simulink model "ccp_slave_demo"  (Simulink 7.3)
settings: Solver=ode3  SolverMode=SingleTasking  StartTime=0.0  StopTime=10.0  RelTol=1e-3
PreLoadFcn:
  | waijung.modelPreload; % Required for working with Waijung Blockset. Do not remove.
undefined symbols (not defined in the file): LQFP48, STM32F072CB
libraries: simulink x216, waijung_soft_i2c_lib x28, waijung_addon_module x12, stm32f0_flash_lib x10, stm32f0_can_lib x3, stm32f0_reset_lib x1, waijung_crc_lib x1, stm32f0_device_config_lib x1
(part 4 of 6)

== system ccp_slave_demo/CCP Handler/Command Processing/BUILD_CHKSUM/BUILD_CHKSUM Handler/Block Size ==
  In1 : Inport
  In2 : Inport  Port=2
  In3 : Inport  Port=3
  In4 : Inport  Port=4
  Bitwise Operator : simulink/Logic and Bit Operations/Bitwise Operator  logicop=OR  UseBitMask=off  NumInputPorts=4  BitMask=bin2dec('11011001')  BitMaskRealWorld=Stored Integer
  Data Type Conversion{1..4} (4 alike) : DataTypeConversion  OutDataTypeMode=uint32  OutDataType=fixdt(1, 16)  OutScaling=2^0  OutDataTypeStr=uint32
  Shift Arithmetic : simulink/Logic and Bit Operations/Shift Arithmetic  SystemSampleTime=-1  nBitShiftRight=-16  nBinPtShiftRight=0
  Shift Arithmetic1 : simulink/Logic and Bit Operations/Shift Arithmetic  SystemSampleTime=-1  nBitShiftRight=-8  nBinPtShiftRight=0
  Shift Arithmetic3 : simulink/Logic and Bit Operations/Shift Arithmetic  SystemSampleTime=-1  nBitShiftRight=-24  nBinPtShiftRight=0
  Size : Outport
  wires:
  In1/1 -> Data Type Conversion1/1
  In2/1 -> Data Type Conversion2/1
  In3/1 -> Data Type Conversion3/1
  In4/1 -> Data Type Conversion4/1
  Data Type Conversion2/1 -> Shift Arithmetic/1
  Data Type Conversion3/1 -> Shift Arithmetic1/1
  Data Type Conversion4/1 -> Bitwise Operator/4
  Data Type Conversion1/1 -> Shift Arithmetic3/1
  Shift Arithmetic/1 -> Bitwise Operator/2
  Shift Arithmetic1/1 -> Bitwise Operator/3
  Bitwise Operator/1 -> Size/1
  Shift Arithmetic3/1 -> Bitwise Operator/1

== system ccp_slave_demo/CCP Handler/Command Processing/BUILD_CHKSUM/BUILD_CHKSUM Handler/Subsystem ==
  In2 : Inport
  In3 : Inport  Port=2
  Enable : EnablePort
  While Iterator Subsystem : Subsystem  TreatAsAtomicUnit=on
  Out2 : Outport
  wires:
  In2/1 -> While Iterator Subsystem/1(Address)
  In3/1 -> While Iterator Subsystem/2(Size)
  While Iterator Subsystem/1(CRC) -> Out2/1

== system ccp_slave_demo/CCP Handler/Command Processing/BUILD_CHKSUM/BUILD_CHKSUM Handler/Subsystem1 ==
  In1 : Inport
  Bitwise Operator{1..4} (4 alike) : simulink/Logic and Bit Operations/Bitwise Operator  logicop=AND  UseBitMask=on  BitMask=255  BitMaskRealWorld=Stored Integer
  Data Type Conversion{,1..3} (4 alike) : DataTypeConversion  OutDataTypeMode=uint8  OutDataType=fixdt(1, 16)  OutScaling=2^0  OutDataTypeStr=uint8
  Shift Arithmetic : simulink/Logic and Bit Operations/Shift Arithmetic  SystemSampleTime=-1  nBitShiftRight=16  nBinPtShiftRight=0
  Shift Arithmetic1 : simulink/Logic and Bit Operations/Shift Arithmetic  SystemSampleTime=-1  nBitShiftRight=8  nBinPtShiftRight=0
  Shift Arithmetic4 : simulink/Logic and Bit Operations/Shift Arithmetic  SystemSampleTime=-1  nBitShiftRight=24  nBinPtShiftRight=0
  Out1 : Outport
  Out2 : Outport  Port=2
  Out3 : Outport  Port=3
  Out4 : Outport  Port=4
  wires:
  Shift Arithmetic/1 -> Bitwise Operator1/1
  Shift Arithmetic1/1 -> Bitwise Operator2/1
  Bitwise Operator4/1 -> Data Type Conversion/1
  Bitwise Operator1/1 -> Data Type Conversion1/1
  Bitwise Operator2/1 -> Data Type Conversion2/1
  Bitwise Operator3/1 -> Data Type Conversion3/1
  In1/1 -> Shift Arithmetic/1, Shift Arithmetic1/1, Bitwise Operator3/1, Shift Arithmetic4/1
  Data Type Conversion/1 -> Out1/1
  Data Type Conversion1/1 -> Out2/1
  Data Type Conversion2/1 -> Out3/1
  Data Type Conversion3/1 -> Out4/1
  Shift Arithmetic4/1 -> Bitwise Operator4/1

== system ccp_slave_demo/CCP Handler/Command Processing/CLEAR_MEMORY/CLEAR_MEMORY Handler/Block Size ==
  In1 : Inport
  In2 : Inport  Port=2
  In3 : Inport  Port=3
  In4 : Inport  Port=4
  Bitwise Operator : simulink/Logic and Bit Operations/Bitwise Operator  logicop=OR  UseBitMask=off  NumInputPorts=4  BitMask=bin2dec('11011001')  BitMaskRealWorld=Stored Integer
  Data Type Conversion{1..4} (4 alike) : DataTypeConversion  OutDataTypeMode=uint32  OutDataType=fixdt(1, 16)  OutScaling=2^0  OutDataTypeStr=uint32
  Shift Arithmetic : simulink/Logic and Bit Operations/Shift Arithmetic  SystemSampleTime=-1  nBitShiftRight=-16  nBinPtShiftRight=0
  Shift Arithmetic1 : simulink/Logic and Bit Operations/Shift Arithmetic  SystemSampleTime=-1  nBitShiftRight=-8  nBinPtShiftRight=0
  Shift Arithmetic3 : simulink/Logic and Bit Operations/Shift Arithmetic  SystemSampleTime=-1  nBitShiftRight=-24  nBinPtShiftRight=0
  Size : Outport
  wires:
  In1/1 -> Data Type Conversion1/1
  In2/1 -> Data Type Conversion2/1
  In3/1 -> Data Type Conversion3/1
  In4/1 -> Data Type Conversion4/1
  Data Type Conversion2/1 -> Shift Arithmetic/1
  Data Type Conversion3/1 -> Shift Arithmetic1/1
  Data Type Conversion4/1 -> Bitwise Operator/4
  Data Type Conversion1/1 -> Shift Arithmetic3/1
  Shift Arithmetic/1 -> Bitwise Operator/2
  Shift Arithmetic1/1 -> Bitwise Operator/3
  Bitwise Operator/1 -> Size/1
  Shift Arithmetic3/1 -> Bitwise Operator/1

== system ccp_slave_demo/CCP Handler/Command Processing/CLEAR_MEMORY/CLEAR_MEMORY Handler/Flash Erase ==
  Address : Inport
  Size : Inport  Port=2
  Enable : EnablePort
  Terminator4 : Terminator
  While Iterator Subsystem : Subsystem  TreatAsAtomicUnit=on
  wires:
  While Iterator Subsystem/1(Sta) -> Terminator4/1
  Address/1 -> While Iterator Subsystem/1(Address)
  Size/1 -> While Iterator Subsystem/2(Size)

== system ccp_slave_demo/CCP Handler/Command Processing/DNLOAD/DNLOAD_6/DOWNLOAD/DOWNLOAD_6 Handler/Subsystem1 ==
  In1 : Inport
  Bitwise Operator{1..4} (4 alike) : simulink/Logic and Bit Operations/Bitwise Operator  logicop=AND  UseBitMask=on  BitMask=255  BitMaskRealWorld=Stored Integer
  Data Type Conversion{,1..3} (4 alike) : DataTypeConversion  OutDataTypeMode=uint8  OutDataType=fixdt(1, 16)  OutScaling=2^0  OutDataTypeStr=uint8
  Shift Arithmetic : simulink/Logic and Bit Operations/Shift Arithmetic  SystemSampleTime=-1  nBitShiftRight=16  nBinPtShiftRight=0
  Shift Arithmetic1 : simulink/Logic and Bit Operations/Shift Arithmetic  SystemSampleTime=-1  nBitShiftRight=8  nBinPtShiftRight=0
  Shift Arithmetic3 : simulink/Logic and Bit Operations/Shift Arithmetic  SystemSampleTime=-1  nBitShiftRight=24  nBinPtShiftRight=0
  Out1 : Outport
  Out2 : Outport  Port=2
  Out3 : Outport  Port=3
  Out4 : Outport  Port=4
  wires:
  Shift Arithmetic/1 -> Bitwise Operator1/1
  Shift Arithmetic1/1 -> Bitwise Operator2/1
  Bitwise Operator4/1 -> Data Type Conversion/1
  Bitwise Operator1/1 -> Data Type Conversion1/1
  Bitwise Operator2/1 -> Data Type Conversion2/1
  Bitwise Operator3/1 -> Data Type Conversion3/1
  In1/1 -> Shift Arithmetic/1, Shift Arithmetic1/1, Bitwise Operator3/1, Shift Arithmetic3/1
  Data Type Conversion/1 -> Out1/1
  Data Type Conversion1/1 -> Out2/1
  Data Type Conversion2/1 -> Out3/1
  Data Type Conversion3/1 -> Out4/1
  Shift Arithmetic3/1 -> Bitwise Operator4/1

== system ccp_slave_demo/CCP Handler/Command Processing/DNLOAD/DNLOAD_6/DOWNLOAD/DOWNLOAD_6 Handler/Write DOWNLOAD ==
  Offset : Inport
  Data : Inport  Port=2
  Size : Inport  Port=3
  Enable : EnablePort
  Volatile Data Array Write : waijung_addon_module/Data Storage/Volatile Data Array Write  conf=Write  specificaddress=off  storagename=CONTROL  memoryaddress=hex2dec('64000000')  storagetype=uint8  datasize=120*160*3  varname=VolatileDataArray_CONTROL  datatype=uint8  datacount=5  variablesize=on  portpinstr=0  sampletime=inf  blockid=CCPHandlerCommandProcessingDNLOADDNLOAD_6DOWNLOADDOWNLOAD_6HandlerWriteDOWNLOADVolatileDataArrayWrite  inputporttype=[7 3 7]  inputportwidth=[1 5 1 ]  inputportlabel={'Offset', 'Data','Size'}  outputporttype=[]  outputportwidth=[]  outputportlabel={}  compat=0  optionstring="[\"CONTROL\",\"uint8\",\"256\",\"VolatileDataArray_CONTROL\",\"uint8_t\",\"uint8\",\"uint8_t\",\"5\",\"Param1\"]"
  wires:
  Size/1 -> Volatile Data Array Write/3
  Offset/1 -> Volatile Data Array Write/1
  Data/1 -> Volatile Data Array Write/2

== system ccp_slave_demo/CCP Handler/Command Processing/DNLOAD/DNLOAD_6/DOWNLOAD/DOWNLOAD_6 Handler/Write DOWNLOAD_6 ==
  Offset : Inport
  Data : Inport  Port=2
  Enable : EnablePort
  Volatile Data Array Write : waijung_addon_module/Data Storage/Volatile Data Array Write  conf=Write  specificaddress=off  storagename=CONTROL  memoryaddress=hex2dec('64000000')  storagetype=uint8  datasize=120*160*3  varname=VolatileDataArray_CONTROL  datatype=uint8  datacount=6  variablesize=off  portpinstr=0  sampletime=inf  blockid=CCPHandlerCommandProcessingDNLOADDNLOAD_6DOWNLOADDOWNLOAD_6HandlerWriteDOWNLOAD_6VolatileDataArrayWrite  inputporttype=[7 3]  inputportwidth=[1 6]  inputportlabel={'Offset', 'Data'}  outputporttype=[]  outputportwidth=[]  outputportlabel={}  compat=0  optionstring="[\"CONTROL\",\"uint8\",\"256\",\"VolatileDataArray_CONTROL\",\"uint8_t\",\"uint8\",\"uint8_t\",\"6\",\"Param1\"]"
  wires:
  Data/1 -> Volatile Data Array Write/2
  Offset/1 -> Volatile Data Array Write/1

== system ccp_slave_demo/CCP Handler/Command Processing/PROGRAM/ PROGRAM_6/PROGRAM/PROGRAM_6 Handler/EEPROM Program ==
  Offset : Inport
  Data(6) : Inport  Port=2
  Enable : EnablePort
  Compare To Constant : simulink/Logic and Bit Operations/Compare To Constant  SystemSampleTime=-1  relop===  const=1  LogicOutDataTypeMode=uint8  ZeroCross=off
  Compare To Constant1 : simulink/Logic and Bit Operations/Compare To Constant  SystemSampleTime=-1  relop===  const=2  LogicOutDataTypeMode=uint8  ZeroCross=off
  Compare To Constant2 : simulink/Logic and Bit Operations/Compare To Constant  SystemSampleTime=-1  relop===  const=3  LogicOutDataTypeMode=uint8  ZeroCross=off
  Compare To Constant3 : simulink/Logic and Bit Operations/Compare To Constant  SystemSampleTime=-1  relop===  const=4  LogicOutDataTypeMode=uint8  ZeroCross=off
  Compare To Constant4 : simulink/Logic and Bit Operations/Compare To Constant  SystemSampleTime=-1  relop===  const=5  LogicOutDataTypeMode=uint8  ZeroCross=off
  Constant2 : Constant  Value=hex2dec('A0')  OutDataTypeMode=uint8  OutDataType=fixdt(1, 16)  OutScaling=2^0  OutDataTypeStr=uint8
  Data Type Conversion : DataTypeConversion  OutDataType=fixdt(1, 16)  OutScaling=2^0
  Demux : Demux  Outputs=6
  Logical Operator{,1..4} (5 alike) : Logic  AllPortsSameDT=off  OutDataTypeMode=boolean  LogicDataType=fixdt(0, 8)  OutDataTypeStr=boolean
  Logical Operator5 : Logic  Operator=OR  Inputs=5  AllPortsSameDT=off  OutDataTypeMode=boolean  LogicDataType=fixdt(0, 8)  OutDataTypeStr=boolean
  Subsystem : Subsystem
  Subsystem1 : Subsystem
  Subsystem2 : Subsystem
  Subsystem3 : Subsystem
  Subsystem4 : Subsystem
  Success : Outport  OutDataType=fixdt(1, 16)  OutScaling=2^0
  wires:
  Data(6)/1 -> Demux/1
  Offset/1 -> Data Type Conversion/1
  Constant2/1 -> Subsystem/1(SlaveAddr), Subsystem1/1(SlaveAddr), Subsystem2/1(SlaveAddr), Subsystem3/1(SlaveAddr), Subsystem4/1(SlaveAddr)
  Data Type Conversion/1 -> Subsystem/2(Offset), Subsystem1/2(Offset), Subsystem2/2(Offset), Subsystem3/2(Offset), Subsystem4/2(Offset)
  Demux/2 -> Subsystem/3(D0), Subsystem1/3(D0), Subsystem2/3(D0), Subsystem3/3(D0), Subsystem4/3(D0)
  Demux/1 -> Compare To Constant/1, Compare To Constant1/1, Compare To Constant2/1, Compare To Constant3/1, Compare To Constant4/1
  Compare To Constant/1 -> Subsystem/Enable, Logical Operator/1
  Compare To Constant1/1 -> Subsystem1/Enable, Logical Operator1/1
  Demux/3 -> Subsystem1/4(D1), Subsystem2/4(D1), Subsystem3/4(D1), Subsystem4/4(D1)
  Compare To Constant2/1 -> Subsystem2/Enable, Logical Operator2/1
  Demux/4 -> Subsystem2/5(D2), Subsystem3/5(D2), Subsystem4/5(D2)
  Compare To Constant3/1 -> Subsystem3/Enable, Logical Operator3/1
  Demux/5 -> Subsystem3/6(D3), Subsystem4/6(D3)
  Demux/6 -> Subsystem4/7(D4)
  Compare To Constant4/1 -> Subsystem4/Enable, Logical Operator4/1
  Subsystem/1(Success) -> Logical Operator/2
  Subsystem1/1(Success) -> Logical Operator1/2
  Subsystem2/1(Success) -> Logical Operator2/2
  Subsystem3/1(Success) -> Logical Operator3/2
  Subsystem4/1(Success) -> Logical Operator4/2
  Logical Operator/1 -> Logical Operator5/1
  Logical Operator4/1 -> Logical Operator5/5
  Logical Operator3/1 -> Logical Operator5/4
  Logical Operator2/1 -> Logical Operator5/3
  Logical Operator1/1 -> Logical Operator5/2
  Logical Operator5/1 -> Success/1

== system ccp_slave_demo/CCP Handler/Command Processing/PROGRAM/ PROGRAM_6/PROGRAM/PROGRAM_6 Handler/EEPROM Program 6 ==
  Offset : Inport
  Data(6) : Inport  Port=2
  Enable : EnablePort
  Constant2 : Constant  Value=hex2dec('A0')  OutDataTypeMode=uint8  OutDataType=fixdt(1, 16)  OutScaling=2^0  OutDataTypeStr=uint8
  Data Type Conversion : DataTypeConversion  OutDataType=fixdt(1, 16)  OutScaling=2^0
  Demux : Demux  Outputs=6
  MEM_FLASH : simulink/Logic and Bit Operations/Compare To Constant  SystemSampleTime=-1  relop===  const=0  LogicOutDataTypeMode=uint8  ZeroCross=off
  Soft I2C Master Read/Write : waijung_soft_i2c_lib/Soft I2C Master Read//Write  conf=ReadWrite  targetname=stm32f0  module=1  transfer=Blocking  clk=100  timeout=25  sdapins={'A4','A6'}  sclpins='A5'  writecount=7  readcount=0  waittime=5  forcestop=off  portpinstr=0  sampletime=inf  blockid=CCPHandlerCommandProcessingPROGRAMPROGRAM_6PROGRAMPROGRAM_6HandlerEEPROMProgram6SoftI2CMasterReadWrite  inputporttype=[3 3 3 3 3 3 3 3]  inputportwidth=[]  inputportlabel={'SlvAddr' 'Wr0 (uint8)' 'Wr1 (uint8)' 'Wr2 (uint8)' 'Wr3 (uint8)' 'Wr4 (uint8)' 'Wr5 (uint8)' 'Wr6 (uint8)'}  outputporttype=[3]  outputportwidth=[1]  outputportlabel={'Status'}  compat=0  optionstring="[\"1\",\"7\",\"0\",\"5\",\"off\",\"1\"]"
  Success : Outport  OutDataType=fixdt(1, 16)  OutScaling=2^0
  wires:
  Data(6)/1 -> Demux/1
  Constant2/1 -> Soft I2C Master Read/Write/1
  Offset/1 -> Data Type Conversion/1
  Data Type Conversion/1 -> Soft I2C Master Read/Write/2
  Demux/1 -> Soft I2C Master Read/Write/3
  Demux/2 -> Soft I2C Master Read/Write/4
  Demux/3 -> Soft I2C Master Read/Write/5
  Demux/4 -> Soft I2C Master Read/Write/6
  Demux/5 -> Soft I2C Master Read/Write/7
  Demux/6 -> Soft I2C Master Read/Write/8
  Soft I2C Master Read/Write/1 -> MEM_FLASH/1
  MEM_FLASH/1 -> Success/1

== system ccp_slave_demo/CCP Handler/Command Processing/PROGRAM/ PROGRAM_6/PROGRAM/PROGRAM_6 Handler/Flash Program ==
  Offset : Inport
  Data(6) : Inport  Port=2
  Enable : EnablePort
  Compare To Constant : simulink/Logic and Bit Operations/Compare To Constant  SystemSampleTime=-1  relop===  const=2  LogicOutDataTypeMode=uint8  ZeroCross=off
  Compare To Constant1 : simulink/Logic and Bit Operations/Compare To Constant  SystemSampleTime=-1  relop===  const=4  LogicOutDataTypeMode=uint8  ZeroCross=off
  Demux : Demux  Outputs=6
  Logical Operator1 : Logic  AllPortsSameDT=off  OutDataTypeMode=boolean  LogicDataType=fixdt(0, 8)  OutDataTypeStr=boolean
  Logical Operator2 : Logic  Operator=OR  AllPortsSameDT=off  OutDataTypeMode=boolean  LogicDataType=fixdt(0, 8)  OutDataTypeStr=boolean
  Logical Operator4 : Logic  AllPortsSameDT=off  OutDataTypeMode=boolean  LogicDataType=fixdt(0, 8)  OutDataTypeStr=boolean
  Subsystem : Subsystem
  Subsystem1 : Subsystem
  Terminator1 : Terminator
  UART Tx : S-Function  FunctionName=stm32f0_uart  Parameters=conf,inputporttype,inputportwidth,outputporttype,outputportwidth,asciiheader,optionstring,headerstring,terminatorstring,asciidatatypestring,sampletime,blockid  EnableBusSupport=off  mask(stm32f0_uart){conf=Tx, uartmodule=1, baudrate=115200, databits=8, parity=No, stopbit=1, remaptxpin=A9, remaprxpin=A10, flowcontrol=None, remapctspin=Not used, remaprtspin=Not used, advanceoptions=off, rxbuffersize=64, txbuffersize=64, transfer=Non-Blocking, packetmode=Ascii, binheader='7E 7E', binterminator='03 03', porttype_double=0, porttype_single=0, porttype_int8=0, porttype_uint8=0, porttype_int16=0, porttype_uint16=0, porttype_int32=0, porttype_uint32=2, asciiformat='Program6: 0x%X, sta=%u,%u', rx_asciiterminator=CR (0x0D - "\r"), tx_asciiterminator=CRLF (0x0D 0x0A - "\r\n"), storagename=<empty>, varname=, asciiheader=Program6: 0x%X, sta=%u,%u\r\n, sampletime=inf, enablecustomportlabel=off, cinputportlabel=de, coutputportlabel=fff,ff,sdfsd, portpinstr=0, blockid=CCPHandlerCommandProcessingPROGRAMPROGRAM_6PROGRAMPROGRAM_6HandlerFlashProgramUARTTx, inputporttype=[ -1 -1 -1], inputportwidth=[], inputportlabel={ '%X' '%u' '%u'}, outputporttype=[], outputportwidth=[], outputportlabel={}, compat=0, optionstring=["1", "1", "A", "9", "1", "A", "10", "0", "*", "*", "0", "*", "*", "1", "1", "", "", "115200", "8", "No", "1", "None", "3", "2", "64", "64", "Ascii", "Non-Blocking", ""], headerstring=[], terminatorstring=["13","10"], asciidatatypestring=["uint32_t","uint32_t","uint32_t"], lastmodule=1}
      mask prompts: conf "Configuration"; uartmodule "UART Module"; baudrate "Baud rate (bps)"; databits "Data bits"; stopbit "Stop bit"; remaptxpin "Tx pin"; remaprxpin "Rx pin"; flowcontrol "Hardware flow control"; remapctspin "HW Flow control, CTS Pin"; remaprtspin "HW Flow control, RTS Pin"; advanceoptions "Advance options"; rxbuffersize "Rx buffer size (bytes)"; txbuffersize "Tx buffer size (bytes)"; packetmode "Packet mode"; binheader "Binary header (example: '7E 7E')"; binterminator "Binary terminator (example: '03 03')"; porttype_double "Number of data port, type DOUBLE"; porttype_single "Number of data port, type SINGLE"; porttype_int8 "Number of data port, type INT8"; porttype_uint8 "Number of data port, type UINT8"; porttype_int16 "Number of data port, type INT16"; porttype_uint16 "Number of data port, type UINT16"; porttype_int32 "Number of data port, type INT32"; porttype_uint32 "Number of data port, type UINT32"; asciiformat "Ascii format"; rx_asciiterminator "End of packet"; tx_asciiterminator "End of packet"; storagename "Buffer"; varname "Var name"; asciiheader "Ascii header (printf format)"; sampletime "Sample time (sec)"; enablecustomportlabel "Enable custom port labels (Ex. In1, In2, In3)"; cinputportlabel "Custom input port labels (Ex. In1, In2, In3)"; coutputportlabel "Custom output port labels (Ex. Out1, Out2, Out3)"; portpinstr "Port Pin String"; blockid "Block ID"; inputporttype "Input Port Type"; inputportwidth "Input Port Width"; inputportlabel "Input Port Label"; outputporttype "Output Port Type"; outputportwidth "Output Port Width"; outputportlabel "Output port label"; compat "Compatibility (Reserved for future use)"; optionstring "String(s) to be passed to TLC"; lastmodule "Last module selected"
      mask help:
      | UART Module
      |  - Select module corresponding to "UART Setup" block.
      | Transfer
      |  - Blocking: after write DMA buffer, the block wait until buffer empty.
      |  - Non-Blocking: the block will not wait for buffer empty.
      | Packet mode:
      |  - Ascii: sending data is ascii, Ascii format + End of packet.
      |  - Binary: sending data is binary format, Header + Data + Terminator
      |  - String Buffer: Volatile Data Storage variable name as sending data.
      | Ascii format:
      |  - %U, %I, %D, %O, %X, %u, %i, %d, %o, %x: Uint32
      |  - %E, %G, %F, %e, %g, %f: Single
      |  - %C, %c: Int8
      |  - %S, %s: (char *), this port is output of Volatile Data Storage Read block, which data type is string.
      mask init:
      | stm32f0_uart_callback('init');
      mask Help: web(fullfile(waijungdocroot,'stm32f0_uart_tx.htm'), '-browser')
      mask StyleString: popup(Setup|Tx|Rx),popup(1|2|3|4),edit,popup(8),popup(No|Odd|Even),popup(0.5|1|1.5|2),popup(Not used|A9|B6),popup(Not used|A10|B7),popup(None|RTS|CTS|RTS/CTS),popup(Not used|A11),popup(Not used|A12),checkbox,popup(16|32|64|128|256|512),popup(16|32|64|128|256|512),popup(Blocking|Non-Blocking),popup(Ascii|Binary|String Buffer),edit,edit,edit,edit,edit,edit,edit,edit,edit,edit,edit,popup(CR (0x0D - "\r")|LF (0x0A - "\n")|CRLF (0x0D 0x0A - "\r\n")),popup(CR (0x0D - "\r")|LF (0x0A - "\n")|CRLF (0x0D 0x0A - "\r\n")|None),popup(<empty>),edit,edit,edit,checkbox,edit,edit,edit,edit,edit,edit,edit,edit,edit,edit,edit,edit,edit,edit,edit,edit
      mask CallbackString: stm32f0_uart_callback('conf');|stm32f0_uart_callback('uartmodule');|||||||stm32f0_uart_callback('flowcontrol');|||stm32f0_uart_callback('advanceoptions');|||stm32f0_uart_callback('conf');|stm32f0_uart_callback('conf');|stm32f0_uart_callback('binheader');|stm32f0_uart_callback('binterminator');|||||||||stm32f0_uart_callback('asciiformat');|||stm32f0_uart_callback('storagename');|||stm32f0_uart_callback('sampletime');|stm32f0_uart_callback('enablecustomportlabel');|stm32f0_uart_callback('conf');|stm32f0_uart_callback('conf');||stm32f0_uart_callback('blockid');||||||||||||
      mask Display: text(0.95, 0.5, 'Module: USART1_Tx\nPacket: Ascii\nTransfer: Non-Blocking\nTs (sec): 0.01','ver','middle','hor','right'); port_label('input', 1,'%X'); port_label('input', 2,'%u'); port_label('input', 3,'%u');
  Success : Outport  OutDataType=fixdt(1, 16)  OutScaling=2^0
  wires:
  Data(6)/1 -> Demux/1
  Offset/1 -> Subsystem/1(Addr), Subsystem1/1(Addr), UART Tx/1
  Demux/2 -> Subsystem/2(In3), Subsystem1/2(In3)
  Demux/3 -> Subsystem/3(In4), Subsystem1/3(In4)
  Demux/1 -> Compare To Constant/1, Compare To Constant1/1
  Compare To Constant/1 -> Subsystem/Enable, Logical Operator4/1
  Compare To Constant1/1 -> Subsystem1/Enable, Logical Operator1/1
  Demux/4 -> Subsystem1/4(In1)
  Demux/5 -> Subsystem1/5(In2)
  Demux/6 -> Terminator1/1
  Subsystem/1(Success) -> Logical Operator4/2
  Subsystem1/1(Success) -> Logical Operator1/2
  Logical Operator4/1 -> Logical Operator2/1, UART Tx/2
  Logical Operator1/1 -> Logical Operator2/2, UART Tx/3
  Logical Operator2/1 -> Success/1

== system ccp_slave_demo/CCP Handler/Command Processing/PROGRAM/ PROGRAM_6/PROGRAM/PROGRAM_6 Handler/Flash Program 6 ==
  Offset : Inport
  Data(6) : Inport  Port=2
  Enable : EnablePort
  Add : Sum  OutDataType=fixdt(1, 16)  OutScaling=2^-10
  Constant : Constant  Value=2  OutDataTypeMode=uint32  OutDataType=fixdt(1, 16)  OutScaling=2^0  OutDataTypeStr=uint32
  Demux2 : Demux  Outputs=6
  FLASH Write : stm32f0_flash_lib/FLASH Write  conf=Write  startaddress=0x8011000  pagesize=2k  datatype=uint16  enablestatus=on  sampletime=inf  filename='ccp_slave_demo.flash'  enablecustomportlabel=off  cinputportlabel=0  portpinstr=0  blockid=CCPHandlerCommandProcessingPROGRAMPROGRAM_6PROGRAMPROGRAM_6HandlerFlashProgram6FLASHWrite  inputporttype=[7 5]  inputportwidth=[]  inputportlabel={'Offset','Data (uint16)'}  outputporttype=[3]  outputportwidth=[]  outputportlabel={'Status'}  compat=0  optionstring="[\"8011000\",\"0\"]"
  FLASH Write1 : stm32f0_flash_lib/FLASH Write  conf=Write  startaddress=0x8011000  pagesize=2k  datatype=uint32  enablestatus=on  sampletime=inf  filename='ccp_slave_demo.flash'  enablecustomportlabel=off  cinputportlabel=0  portpinstr=0  blockid=CCPHandlerCommandProcessingPROGRAMPROGRAM_6PROGRAMPROGRAM_6HandlerFlashProgram6FLASHWrite1  inputporttype=[7 7]  inputportwidth=[]  inputportlabel={'Offset','Data (uint32)'}  outputporttype=[3]  outputportwidth=[]  outputportlabel={'Status'}  compat=0  optionstring="[\"8011000\",\"0\"]"
  FLASH_COMPLETE : simulink/Logic and Bit Operations/Compare To Constant  SystemSampleTime=-1  relop===  const=4  LogicOutDataTypeMode=uint8  ZeroCross=off
  FLASH_COMPLETE1 : simulink/Logic and Bit Operations/Compare To Constant  SystemSampleTime=-1  relop===  const=4  LogicOutDataTypeMode=uint8  ZeroCross=off
  Logical Operator : Logic  AllPortsSameDT=off  OutDataTypeMode=boolean  LogicDataType=fixdt(0, 8)  OutDataTypeStr=boolean
  Subsystem : Subsystem
  Subsystem1 : Subsystem
  UART Tx : S-Function  FunctionName=stm32f0_uart  Parameters=conf,inputporttype,inputportwidth,outputporttype,outputportwidth,asciiheader,optionstring,headerstring,terminatorstring,asciidatatypestring,sampletime,blockid  EnableBusSupport=off  mask(stm32f0_uart){conf=Tx, uartmodule=1, baudrate=115200, databits=8, parity=No, stopbit=1, remaptxpin=A9, remaprxpin=A10, flowcontrol=None, remapctspin=Not used, remaprtspin=Not used, advanceoptions=off, rxbuffersize=64, txbuffersize=64, transfer=Non-Blocking, packetmode=Ascii, binheader='7E 7E', binterminator='03 03', porttype_double=0, porttype_single=0, porttype_int8=0, porttype_uint8=0, porttype_int16=0, porttype_uint16=0, porttype_int32=0, porttype_uint32=2, asciiformat='Program6: 0x%X, sta=%u,%u', rx_asciiterminator=CR (0x0D - "\r"), tx_asciiterminator=CRLF (0x0D 0x0A - "\r\n"), storagename=<empty>, varname=, asciiheader=Program6: 0x%X, sta=%u,%u\r\n, sampletime=inf, enablecustomportlabel=off, cinputportlabel=de, coutputportlabel=fff,ff,sdfsd, portpinstr=0, blockid=CCPHandlerCommandProcessingPROGRAMPROGRAM_6PROGRAMPROGRAM_6HandlerFlashProgram6UARTTx, inputporttype=[ -1 -1 -1], inputportwidth=[], inputportlabel={ '%X' '%u' '%u'}, outputporttype=[], outputportwidth=[], outputportlabel={}, compat=0, optionstring=["1", "1", "A", "9", "1", "A", "10", "0", "*", "*", "0", "*", "*", "1", "1", "", "", "115200", "8", "No", "1", "None", "3", "2", "64", "64", "Ascii", "Non-Blocking", ""], headerstring=[], terminatorstring=["13","10"], asciidatatypestring=["uint32_t","uint32_t","uint32_t"], lastmodule=1}
      mask prompts: conf "Configuration"; uartmodule "UART Module"; baudrate "Baud rate (bps)"; databits "Data bits"; stopbit "Stop bit"; remaptxpin "Tx pin"; remaprxpin "Rx pin"; flowcontrol "Hardware flow control"; remapctspin "HW Flow control, CTS Pin"; remaprtspin "HW Flow control, RTS Pin"; advanceoptions "Advance options"; rxbuffersize "Rx buffer size (bytes)"; txbuffersize "Tx buffer size (bytes)"; packetmode "Packet mode"; binheader "Binary header (example: '7E 7E')"; binterminator "Binary terminator (example: '03 03')"; porttype_double "Number of data port, type DOUBLE"; porttype_single "Number of data port, type SINGLE"; porttype_int8 "Number of data port, type INT8"; porttype_uint8 "Number of data port, type UINT8"; porttype_int16 "Number of data port, type INT16"; porttype_uint16 "Number of data port, type UINT16"; porttype_int32 "Number of data port, type INT32"; porttype_uint32 "Number of data port, type UINT32"; asciiformat "Ascii format"; rx_asciiterminator "End of packet"; tx_asciiterminator "End of packet"; storagename "Buffer"; varname "Var name"; asciiheader "Ascii header (printf format)"; sampletime "Sample time (sec)"; enablecustomportlabel "Enable custom port labels (Ex. In1, In2, In3)"; cinputportlabel "Custom input port labels (Ex. In1, In2, In3)"; coutputportlabel "Custom output port labels (Ex. Out1, Out2, Out3)"; portpinstr "Port Pin String"; blockid "Block ID"; inputporttype "Input Port Type"; inputportwidth "Input Port Width"; inputportlabel "Input Port Label"; outputporttype "Output Port Type"; outputportwidth "Output Port Width"; outputportlabel "Output port label"; compat "Compatibility (Reserved for future use)"; optionstring "String(s) to be passed to TLC"; lastmodule "Last module selected"
      mask help:
      | UART Module
      |  - Select module corresponding to "UART Setup" block.
      | Transfer
      |  - Blocking: after write DMA buffer, the block wait until buffer empty.
      |  - Non-Blocking: the block will not wait for buffer empty.
      | Packet mode:
      |  - Ascii: sending data is ascii, Ascii format + End of packet.
      |  - Binary: sending data is binary format, Header + Data + Terminator
      |  - String Buffer: Volatile Data Storage variable name as sending data.
      | Ascii format:
      |  - %U, %I, %D, %O, %X, %u, %i, %d, %o, %x: Uint32
      |  - %E, %G, %F, %e, %g, %f: Single
      |  - %C, %c: Int8
      |  - %S, %s: (char *), this port is output of Volatile Data Storage Read block, which data type is string.
      mask init:
      | stm32f0_uart_callback('init');
      mask Help: web(fullfile(waijungdocroot,'stm32f0_uart_tx.htm'), '-browser')
      mask StyleString: popup(Setup|Tx|Rx),popup(1|2|3|4),edit,popup(8),popup(No|Odd|Even),popup(0.5|1|1.5|2),popup(Not used|A9|B6),popup(Not used|A10|B7),popup(None|RTS|CTS|RTS/CTS),popup(Not used|A11),popup(Not used|A12),checkbox,popup(16|32|64|128|256|512),popup(16|32|64|128|256|512),popup(Blocking|Non-Blocking),popup(Ascii|Binary|String Buffer),edit,edit,edit,edit,edit,edit,edit,edit,edit,edit,edit,popup(CR (0x0D - "\r")|LF (0x0A - "\n")|CRLF (0x0D 0x0A - "\r\n")),popup(CR (0x0D - "\r")|LF (0x0A - "\n")|CRLF (0x0D 0x0A - "\r\n")|None),popup(<empty>),edit,edit,edit,checkbox,edit,edit,edit,edit,edit,edit,edit,edit,edit,edit,edit,edit,edit,edit,edit,edit
      mask CallbackString: stm32f0_uart_callback('conf');|stm32f0_uart_callback('uartmodule');|||||||stm32f0_uart_callback('flowcontrol');|||stm32f0_uart_callback('advanceoptions');|||stm32f0_uart_callback('conf');|stm32f0_uart_callback('conf');|stm32f0_uart_callback('binheader');|stm32f0_uart_callback('binterminator');|||||||||stm32f0_uart_callback('asciiformat');|||stm32f0_uart_callback('storagename');|||stm32f0_uart_callback('sampletime');|stm32f0_uart_callback('enablecustomportlabel');|stm32f0_uart_callback('conf');|stm32f0_uart_callback('conf');||stm32f0_uart_callback('blockid');||||||||||||
      mask Display: text(0.95, 0.5, 'Module: USART1_Tx\nPacket: Ascii\nTransfer: Non-Blocking\nTs (sec): 0.01','ver','middle','hor','right'); port_label('input', 1,'%X'); port_label('input', 2,'%u'); port_label('input', 3,'%u');
  Success : Outport  OutDataType=fixdt(1, 16)  OutScaling=2^0
  wires:
  Offset/1 -> FLASH Write/1, Add/1, UART Tx/1
  Data(6)/1 -> Demux2/1
  Demux2/1 -> Subsystem/1(In1)
  Demux2/2 -> Subsystem/2(In2)
  Subsystem/1(Out1) -> FLASH Write/2
  Demux2/3 -> Subsystem1/1(In1)
  Demux2/4 -> Subsystem1/2(In2)
  Demux2/5 -> Subsystem1/3(In3)
  Demux2/6 -> Subsystem1/4(In4)
  Subsystem1/1(Out1) -> FLASH Write1/2
  Add/1 -> FLASH Write1/1
  Constant/1 -> Add/2
  FLASH Write/1 -> FLASH_COMPLETE/1
  FLASH Write1/1 -> FLASH_COMPLETE1/1
  FLASH_COMPLETE/1 -> Logical Operator/1, UART Tx/2
  FLASH_COMPLETE1/1 -> Logical Operator/2, UART Tx/3
  Logical Operator/1 -> Success/1

== system ccp_slave_demo/CCP Handler/Command Processing/PROGRAM/ PROGRAM_6/PROGRAM/PROGRAM_6 Handler/Subsystem1 ==
  In1 : Inport
  Bitwise Operator{1..4} (4 alike) : simulink/Logic and Bit Operations/Bitwise Operator  logicop=AND  UseBitMask=on  BitMask=255  BitMaskRealWorld=Stored Integer
  Data Type Conversion{,1..3} (4 alike) : DataTypeConversion  OutDataTypeMode=uint8  OutDataType=fixdt(1, 16)  OutScaling=2^0  OutDataTypeStr=uint8
  Shift Arithmetic : simulink/Logic and Bit Operations/Shift Arithmetic  SystemSampleTime=-1  nBitShiftRight=16  nBinPtShiftRight=0
  Shift Arithmetic1 : simulink/Logic and Bit Operations/Shift Arithmetic  SystemSampleTime=-1  nBitShiftRight=8  nBinPtShiftRight=0
  Shift Arithmetic3 : simulink/Logic and Bit Operations/Shift Arithmetic  SystemSampleTime=-1  nBitShiftRight=24  nBinPtShiftRight=0
  Out1 : Outport
  Out2 : Outport  Port=2
  Out3 : Outport  Port=3
  Out4 : Outport  Port=4
  wires:
  Shift Arithmetic/1 -> Bitwise Operator1/1
  Shift Arithmetic1/1 -> Bitwise Operator2/1
  Bitwise Operator4/1 -> Data Type Conversion/1
  Bitwise Operator1/1 -> Data Type Conversion1/1
  Bitwise Operator2/1 -> Data Type Conversion2/1
  Bitwise Operator3/1 -> Data Type Conversion3/1
  In1/1 -> Shift Arithmetic/1, Shift Arithmetic1/1, Bitwise Operator3/1, Shift Arithmetic3/1
  Data Type Conversion/1 -> Out1/1
  Data Type Conversion1/1 -> Out2/1
  Data Type Conversion2/1 -> Out3/1
  Data Type Conversion3/1 -> Out4/1
  Shift Arithmetic3/1 -> Bitwise Operator4/1

== system ccp_slave_demo/CCP Handler/Command Processing/SHORT_UP/SHORT_UP Handler/Subsystem ==
  In1 : Inport
  In2 : Inport  Port=2
  In3 : Inport  Port=3
  In4 : Inport  Port=4
  Bitwise Operator : simulink/Logic and Bit Operations/Bitwise Operator  logicop=OR  UseBitMask=off  NumInputPorts=4  BitMask=bin2dec('11011001')  BitMaskRealWorld=Stored Integer
  Data Type Conversion{1..4} (4 alike) : DataTypeConversion  OutDataTypeMode=uint32  OutDataType=fixdt(1, 16)  OutScaling=2^0  OutDataTypeStr=uint32
  Shift Arithmetic : simulink/Logic and Bit Operations/Shift Arithmetic  SystemSampleTime=-1  nBitShiftRight=-24  nBinPtShiftRight=0
  Shift Arithmetic1 : simulink/Logic and Bit Operations/Shift Arithmetic  SystemSampleTime=-1  nBitShiftRight=-16  nBinPtShiftRight=0
  Shift Arithmetic2 : simulink/Logic and Bit Operations/Shift Arithmetic  SystemSampleTime=-1  nBitShiftRight=-8  nBinPtShiftRight=0
  Out1 : Outport
  wires:
  Data Type Conversion1/1 -> Shift Arithmetic/1
  Data Type Conversion2/1 -> Shift Arithmetic1/1
  Data Type Conversion3/1 -> Shift Arithmetic2/1
  Shift Arithmetic/1 -> Bitwise Operator/1
  Data Type Conversion4/1 -> Bitwise Operator/4
  Shift Arithmetic2/1 -> Bitwise Operator/3
  Shift Arithmetic1/1 -> Bitwise Operator/2
  In1/1 -> Data Type Conversion1/1
  Bitwise Operator/1 -> Out1/1
  In2/1 -> Data Type Conversion2/1
  In3/1 -> Data Type Conversion3/1
  In4/1 -> Data Type Conversion4/1

== system ccp_slave_demo/CCP Handler/Command Processing/SHORT_UP/SHORT_UP Handler/UPLOAD ==
  Mem Sector : Inport
  Offset : Inport  Port=2
  Size : Inport  Port=3
  Enable : EnablePort
  Compare To Constant : simulink/Logic and Bit Operations/Compare To Constant  SystemSampleTime=-1  relop===  const=0  LogicOutDataTypeMode=uint8  ZeroCross=off
  Compare To Constant1 : simulink/Logic and Bit Operations/Compare To Constant  SystemSampleTime=-1  relop===  const=1  LogicOutDataTypeMode=uint8  ZeroCross=off
  Compare To Constant2 : simulink/Logic and Bit Operations/Compare To Constant  SystemSampleTime=-1  relop===  const=2  LogicOutDataTypeMode=uint8  ZeroCross=off
  Compare To Constant3 : simulink/Logic and Bit Operations/Compare To Constant  SystemSampleTime=-1  relop===  const=3  LogicOutDataTypeMode=uint8  ZeroCross=off
  Compare To Constant4 : simulink/Logic and Bit Operations/Compare To Constant  SystemSampleTime=-1  relop===  const=4  LogicOutDataTypeMode=uint8  ZeroCross=off
  MEM_EEPROM : Subsystem  TreatAsAtomicUnit=on
  MEM_FLASH : Subsystem  TreatAsAtomicUnit=on
  MEM_RO : Subsystem  TreatAsAtomicUnit=on
  MEM_RW : Subsystem  TreatAsAtomicUnit=on
  Multiport Switch : MultiPortSwitch  Inputs=5  zeroidx=on  OutDataType=fixdt(1, 16)  OutScaling=2^0
  Multiport Switch1 : MultiPortSwitch  Inputs=5  zeroidx=on  OutDataType=fixdt(1, 16)  OutScaling=2^0
  SLAVE_DEVICE_ID : Subsystem  TreatAsAtomicUnit=on
  Valid : Outport  OutDataType=fixdt(1, 16)  OutScaling=2^0  InitialOutput=0
  Out1 : Outport  Port=2  OutDataType=fixdt(1, 16)  OutScaling=2^0  InitialOutput=[0 0 0 0 0]
  wires:
  Mem Sector/1 -> Compare To Constant/1, Compare To Constant1/1, Compare To Constant2/1, Compare To Constant3/1, Compare To Constant4/1, Multiport Switch/1, Multiport Switch1/1
  Compare To Constant/1 -> SLAVE_DEVICE_ID/Enable
  Offset/1 -> SLAVE_DEVICE_ID/1(Offset), MEM_RO/1(Offset), MEM_RW/1(Offset), MEM_FLASH/1(Offset), MEM_EEPROM/1(Offset)
  Size/1 -> SLAVE_DEVICE_ID/2(Size), MEM_RO/2(Size), MEM_RW/2(Size), MEM_FLASH/2(Size), MEM_EEPROM/2(Size)
  Compare To Constant1/1 -> MEM_RO/Enable
  Compare To Constant2/1 -> MEM_RW/Enable
  Compare To Constant3/1 -> MEM_FLASH/Enable
  Compare To Constant4/1 -> MEM_EEPROM/Enable
  SLAVE_DEVICE_ID/1(Valid) -> Multiport Switch/2
  MEM_EEPROM/1(Valid) -> Multiport Switch/6
  MEM_FLASH/1(Valid) -> Multiport Switch/5
  MEM_RW/1(Valid) -> Multiport Switch/4
  MEM_RO/1(Valid) -> Multiport Switch/3
  SLAVE_DEVICE_ID/2(Out1) -> Multiport Switch1/2
  MEM_EEPROM/2(Out1) -> Multiport Switch1/6
  MEM_FLASH/2(Out1) -> Multiport Switch1/5
  MEM_RW/2(Out1) -> Multiport Switch1/4
  MEM_RO/2(Out1) -> Multiport Switch1/3
  Multiport Switch/1 -> Valid/1
  Multiport Switch1/1 -> Out1/1

== system ccp_slave_demo/CCP Handler/Command Processing/SHORT_UP/SHORT_UP Handler/Validate Base Address ==
  ExtAddr : Inport
  PostIncAddr : Inport  Port=2
  Compare To Constant : simulink/Logic and Bit Operations/Compare To Constant  SystemSampleTime=-1  relop=<=  const=4  LogicOutDataTypeMode=uint8  ZeroCross=off
  Demux : Demux  Outputs=2
  INVALID_EXTADDR : Constant  Value=0  OutDataTypeMode=uint8  OutDataType=fixdt(1, 16)  OutScaling=2^0  OutDataTypeStr=uint8
  Interval Test Dynamic : simulink/Logic and Bit Operations/Interval Test Dynamic  SystemSampleTime=-1  IntervalClosedRight=on  IntervalClosedLeft=on  LogicOutDataTypeMode=uint8
  Limit EXT_0 (ID) : Constant  Value=[16 0]  OutDataTypeMode=uint32  OutDataType=fixdt(1, 16)  OutScaling=2^0  OutDataTypeStr=uint32
  Limit EXT_1 (RO) : Constant  Value=[255 0]  OutDataTypeMode=uint32  OutDataType=fixdt(1, 16)  OutScaling=2^0  OutDataTypeStr=uint32
  Limit EXT_2 (RW) : Constant  Value=[255 0]  OutDataTypeMode=uint32  OutDataType=fixdt(1, 16)  OutScaling=2^0  OutDataTypeStr=uint32
  Limit EXT_3 (FLASH) : Constant  Value=[52*1024 0]  OutDataTypeMode=uint32  OutDataType=fixdt(1, 16)  OutScaling=2^0  OutDataTypeStr=uint32
  Limit EXT_4 (EEPROM) : Constant  Value=[255 0]  OutDataTypeMode=uint32  OutDataType=fixdt(1, 16)  OutScaling=2^0  OutDataTypeStr=uint32
  Multiport Switch : MultiPortSwitch  Inputs=5  zeroidx=on  OutDataType=fixdt(1, 16)  OutScaling=2^0
  Saturation : Saturate  UpperLimit=4  LowerLimit=0  OutDataType=fixdt(1, 16)  OutScaling=2^0
  Switch : Switch  Criteria=u2 ~= 0  OutDataType=fixdt(1, 16)  OutScaling=2^0
  ValidAddr : Outport  OutDataType=fixdt(1, 16)  OutScaling=2^0
  wires:
  ExtAddr/1 -> Compare To Constant/1, Saturation/1
  Compare To Constant/1 -> Switch/2
  INVALID_EXTADDR/1 -> Switch/3
  Limit EXT_0 (ID)/1 -> Multiport Switch/2
  Limit EXT_1 (RO)/1 -> Multiport Switch/3
  Limit EXT_2 (RW)/1 -> Multiport Switch/4
  Limit EXT_3 (FLASH)/1 -> Multiport Switch/5
  Limit EXT_4 (EEPROM)/1 -> Multiport Switch/6
  PostIncAddr/1 -> Interval Test Dynamic/2
  Multiport Switch/1 -> Demux/1
  Interval Test Dynamic/1 -> Switch/1
  Switch/1 -> ValidAddr/1
  Demux/1 -> Interval Test Dynamic/1
  Demux/2 -> Interval Test Dynamic/3
  Saturation/1 -> Multiport Switch/1

== system ccp_slave_demo/CCP Handler/Command Processing/UPLOAD/UPLOAD/UPLOAD ==
  Mem Sector : Inport
  Offset : Inport  Port=2
  Size : Inport  Port=3
  Enable : EnablePort
  Compare To Constant : simulink/Logic and Bit Operations/Compare To Constant  SystemSampleTime=-1  relop===  const=0  LogicOutDataTypeMode=uint8  ZeroCross=off
  Compare To Constant1 : simulink/Logic and Bit Operations/Compare To Constant  SystemSampleTime=-1  relop===  const=1  LogicOutDataTypeMode=uint8  ZeroCross=off
  Compare To Constant2 : simulink/Logic and Bit Operations/Compare To Constant  SystemSampleTime=-1  relop===  const=2  LogicOutDataTypeMode=uint8  ZeroCross=off
  Compare To Constant3 : simulink/Logic and Bit Operations/Compare To Constant  SystemSampleTime=-1  relop===  const=3  LogicOutDataTypeMode=uint8  ZeroCross=off
  Compare To Constant4 : simulink/Logic and Bit Operations/Compare To Constant  SystemSampleTime=-1  relop===  const=4  LogicOutDataTypeMode=uint8  ZeroCross=off
  MEM_EEPROM : Subsystem  TreatAsAtomicUnit=on
  MEM_FLASH : Subsystem  TreatAsAtomicUnit=on
  MEM_RO : Subsystem  TreatAsAtomicUnit=on
  MEM_RW : Subsystem  TreatAsAtomicUnit=on
  Multiport Switch : MultiPortSwitch  Inputs=5  zeroidx=on  OutDataType=fixdt(1, 16)  OutScaling=2^0
  Multiport Switch1 : MultiPortSwitch  Inputs=5  zeroidx=on  OutDataType=fixdt(1, 16)  OutScaling=2^0
  SLAVE_DEVICE_ID : Subsystem  TreatAsAtomicUnit=on
  Valid : Outport  OutDataType=fixdt(1, 16)  OutScaling=2^0  InitialOutput=0
  Out1 : Outport  Port=2  OutDataType=fixdt(1, 16)  OutScaling=2^0  InitialOutput=[0 0 0 0 0]
  wires:
  Mem Sector/1 -> Compare To Constant/1, Compare To Constant1/1, Compare To Constant2/1, Compare To Constant3/1, Compare To Constant4/1, Multiport Switch/1, Multiport Switch1/1
  Compare To Constant/1 -> SLAVE_DEVICE_ID/Enable
  Offset/1 -> SLAVE_DEVICE_ID/1(Offset), MEM_RO/1(Offset), MEM_RW/1(Offset), MEM_FLASH/1(Offset), MEM_EEPROM/1(Offset)
  Size/1 -> SLAVE_DEVICE_ID/2(Size), MEM_RO/2(Size), MEM_RW/2(Size), MEM_FLASH/2(Size), MEM_EEPROM/2(Size)
  Compare To Constant1/1 -> MEM_RO/Enable
  Compare To Constant2/1 -> MEM_RW/Enable
  Compare To Constant3/1 -> MEM_FLASH/Enable
  Compare To Constant4/1 -> MEM_EEPROM/Enable
  SLAVE_DEVICE_ID/1(Valid) -> Multiport Switch/2
  MEM_EEPROM/1(Valid) -> Multiport Switch/6
  MEM_FLASH/1(Valid) -> Multiport Switch/5
  MEM_RW/1(Valid) -> Multiport Switch/4
  MEM_RO/1(Valid) -> Multiport Switch/3
  SLAVE_DEVICE_ID/2(Out1) -> Multiport Switch1/2
  MEM_EEPROM/2(Out1) -> Multiport Switch1/6
  MEM_FLASH/2(Out1) -> Multiport Switch1/5
  MEM_RW/2(Out1) -> Multiport Switch1/4
  MEM_RO/2(Out1) -> Multiport Switch1/3
  Multiport Switch/1 -> Valid/1
  Multiport Switch1/1 -> Out1/1

== system ccp_slave_demo/CCP Handler/Command Processing/BUILD_CHKSUM/BUILD_CHKSUM Handler/Subsystem/While Iterator Subsystem ==
  Address : Inport  OutDataType=fixdt(1, 16)  OutScaling=2^0
  Size : Inport  Port=2  OutDataType=fixdt(1, 16)  OutScaling=2^0
  Add : Sum  OutDataType=fixdt(1, 16)  OutScaling=2^-10
  Add1 : Sum  OutDataType=fixdt(1, 16)  OutScaling=2^-10
  Bitwise Operator : simulink/Logic and Bit Operations/Bitwise Operator  logicop=AND  UseBitMask=on  BitMask=hex2dec('01FFFFFF')  BitMaskRealWorld=Stored Integer
  Bitwise Operator1 : simulink/Logic and Bit Operations/Bitwise Operator  logicop=AND  UseBitMask=on  BitMask=hex2dec('0001FFFF')  BitMaskRealWorld=Stored Integer
  Compare To Zero : simulink/Logic and Bit Operations/Compare To Zero  SystemSampleTime=-1  relop===  LogicOutDataTypeMode=uint8  ZeroCross=off
  Initial : Constant  Value=0  OutDataTypeMode=uint32  OutDataType=fixdt(1, 16)  OutScaling=2^0  OutDataTypeStr=uint32
  Initial1 : Constant  Value=hex2dec('FFFFFFFF')  OutDataTypeMode=uint32  OutDataType=fixdt(1, 16)  OutScaling=2^0  OutDataTypeStr=uint32
  Memory : Memory  InheritSampleTime=on  LinearizeMemory=on
  Memory1 : Memory  InheritSampleTime=on  LinearizeMemory=on
  Relational Operator : RelationalOperator  Operator=>  LogicOutDataTypeMode=boolean  LogicDataType=fixdt(0, 8)  OutDataTypeStr=boolean
  Step : Constant  Value=4  OutDataTypeMode=uint32  OutDataType=fixdt(1, 16)  OutScaling=2^0  OutDataTypeStr=uint32
  Subsystem : Subsystem
  Switch : Switch  Criteria=u2 ~= 0  OutDataType=fixdt(1, 16)  OutScaling=2^0
  Switch1 : Switch  Criteria=u2 ~= 0  OutDataType=fixdt(1, 16)  OutScaling=2^0
  While Iterator : WhileIterator  MaxIters=-1  WhileBlockType=do-while
  CRC : Outport  OutDataType=fixdt(1, 16)  OutScaling=2^0
  wires:
  Initial/1 -> Switch/3
  Add1/1 -> Switch/1
  Relational Operator/1 -> Switch/2, While Iterator/1, Subsystem/Enable
  Switch/1 -> Memory/1
  Size/1 -> Relational Operator/1
  Step/1 -> Add1/2
  Add/1 -> Bitwise Operator/1
  Memory/1 -> Add/2, Relational Operator/2, Add1/1, Compare To Zero/1
  Address/1 -> Bitwise Operator1/1
  Compare To Zero/1 -> Switch1/2
  Initial1/1 -> Switch1/1
  Switch1/1 -> Subsystem/1(In1)
  Subsystem/1(Out1) -> Memory1/1, CRC/1
  Memory1/1 -> Switch1/3
  Bitwise Operator/1 -> Subsystem/2(In2)
  Bitwise Operator1/1 -> Add/1

== system ccp_slave_demo/CCP Handler/Command Processing/CLEAR_MEMORY/CLEAR_MEMORY Handler/Flash Erase/While Iterator Subsystem ==
  Address : Inport  OutDataType=fixdt(1, 16)  OutScaling=2^0
  Size : Inport  Port=2  OutDataType=fixdt(1, 16)  OutScaling=2^0
  Add : Sum  OutDataType=fixdt(1, 16)  OutScaling=2^-10
  Add1 : Sum  OutDataType=fixdt(1, 16)  OutScaling=2^-10
  Bitwise Operator : simulink/Logic and Bit Operations/Bitwise Operator  logicop=AND  UseBitMask=on  BitMask=hex2dec('0000FFFF')  BitMaskRealWorld=Stored Integer
  Initial : Constant  Value=0  OutDataTypeMode=uint32  OutDataType=fixdt(1, 16)  OutScaling=2^0  OutDataTypeStr=uint32
  Memory : Memory  InheritSampleTime=on  LinearizeMemory=on
  Relational Operator : RelationalOperator  Operator=>  LogicOutDataTypeMode=boolean  LogicDataType=fixdt(0, 8)  OutDataTypeStr=boolean
  Step : Constant  Value=2048  OutDataTypeMode=uint32  OutDataType=fixdt(1, 16)  OutScaling=2^0  OutDataTypeStr=uint32
  Subsystem : Subsystem
  Switch : Switch  Criteria=u2 ~= 0  OutDataType=fixdt(1, 16)  OutScaling=2^0
  While Iterator : WhileIterator  MaxIters=-1  WhileBlockType=do-while
  Sta : Outport  OutDataType=fixdt(1, 16)  OutScaling=2^0
  wires:
  Bitwise Operator/1 -> Subsystem/1(Address)
  Subsystem/1(Sta) -> Sta/1
  Address/1 -> Add/1
  Memory/1 -> Add1/1, Relational Operator/2, Add/2
  Add/1 -> Bitwise Operator/1
  Step/1 -> Add1/2
  Size/1 -> Relational Operator/1
  Switch/1 -> Memory/1
  Relational Operator/1 -> Switch/2, While Iterator/1, Subsystem/Enable
  Add1/1 -> Switch/1
  Initial/1 -> Switch/3

== system ccp_slave_demo/CCP Handler/Command Processing/PROGRAM/ PROGRAM_6/PROGRAM/PROGRAM_6 Handler/EEPROM Program/Subsystem ==
  SlaveAddr : Inport
  Offset : Inport  Port=2
  D0 : Inport  Port=3
  Enable : EnablePort
  Compare To Zero : simulink/Logic and Bit Operations/Compare To Zero  SystemSampleTime=-1  relop===  LogicOutDataTypeMode=uint8  ZeroCross=off
  Soft I2C Master Read/Write : waijung_soft_i2c_lib/Soft I2C Master Read//Write  conf=ReadWrite  targetname=stm32f0  module=1  transfer=Blocking  clk=100  timeout=25  sdapins={'A4','A6'}  sclpins='A5'  writecount=2  readcount=0  waittime=5  forcestop=off  portpinstr=0  sampletime=inf  blockid=CCPHandlerCommandProcessingPROGRAMPROGRAM_6PROGRAMPROGRAM_6HandlerEEPROMProgramSubsystemSoftI2CMasterReadWrite  inputporttype=[3 3 3]  inputportwidth=[]  inputportlabel={'SlvAddr' 'Wr0 (uint8)' 'Wr1 (uint8)'}  outputporttype=[3]  outputportwidth=[1]  outputportlabel={'Status'}  compat=0  optionstring="[\"1\",\"2\",\"0\",\"5\",\"off\",\"1\"]"
  Success : Outport
  wires:
  SlaveAddr/1 -> Soft I2C Master Read/Write/1
  Offset/1 -> Soft I2C Master Read/Write/2
  Soft I2C Master Read/Write/1 -> Compare To Zero/1
  D0/1 -> Soft I2C Master Read/Write/3
  Compare To Zero/1 -> Success/1

== system ccp_slave_demo/CCP Handler/Command Processing/PROGRAM/ PROGRAM_6/PROGRAM/PROGRAM_6 Handler/EEPROM Program/Subsystem1 ==
  SlaveAddr : Inport
  Offset : Inport  Port=2
  D0 : Inport  Port=3
  D1 : Inport  Port=4
  Enable : EnablePort
  Compare To Zero : simulink/Logic and Bit Operations/Compare To Zero  SystemSampleTime=-1  relop===  LogicOutDataTypeMode=uint8  ZeroCross=off
  Soft I2C Master Read/Write : waijung_soft_i2c_lib/Soft I2C Master Read//Write  conf=ReadWrite  targetname=stm32f0  module=1  transfer=Blocking  clk=100  timeout=25  sdapins={'A4','A6'}  sclpins='A5'  writecount=3  readcount=0  waittime=5  forcestop=off  portpinstr=0  sampletime=inf  blockid=CCPHandlerCommandProcessingPROGRAMPROGRAM_6PROGRAMPROGRAM_6HandlerEEPROMProgramSubsystem1SoftI2CMasterReadWrite  inputporttype=[3 3 3 3]  inputportwidth=[]  inputportlabel={'SlvAddr' 'Wr0 (uint8)' 'Wr1 (uint8)' 'Wr2 (uint8)'}  outputporttype=[3]  outputportwidth=[1]  outputportlabel={'Status'}  compat=0  optionstring="[\"1\",\"3\",\"0\",\"5\",\"off\",\"1\"]"
  Success : Outport
  wires:
  Compare To Zero/1 -> Success/1
  D0/1 -> Soft I2C Master Read/Write/3
  Soft I2C Master Read/Write/1 -> Compare To Zero/1
  Offset/1 -> Soft I2C Master Read/Write/2
  SlaveAddr/1 -> Soft I2C Master Read/Write/1
  D1/1 -> Soft I2C Master Read/Write/4

== system ccp_slave_demo/CCP Handler/Command Processing/PROGRAM/ PROGRAM_6/PROGRAM/PROGRAM_6 Handler/EEPROM Program/Subsystem2 ==
  SlaveAddr : Inport
  Offset : Inport  Port=2
  D0 : Inport  Port=3
  D1 : Inport  Port=4
  D2 : Inport  Port=5
  Enable : EnablePort
  Compare To Zero : simulink/Logic and Bit Operations/Compare To Zero  SystemSampleTime=-1  relop===  LogicOutDataTypeMode=uint8  ZeroCross=off
  Soft I2C Master Read/Write : waijung_soft_i2c_lib/Soft I2C Master Read//Write  conf=ReadWrite  targetname=stm32f0  module=1  transfer=Blocking  clk=100  timeout=25  sdapins={'A4','A6'}  sclpins='A5'  writecount=4  readcount=0  waittime=5  forcestop=off  portpinstr=0  sampletime=inf  blockid=CCPHandlerCommandProcessingPROGRAMPROGRAM_6PROGRAMPROGRAM_6HandlerEEPROMProgramSubsystem2SoftI2CMasterReadWrite  inputporttype=[3 3 3 3 3]  inputportwidth=[]  inputportlabel={'SlvAddr' 'Wr0 (uint8)' 'Wr1 (uint8)' 'Wr2 (uint8)' 'Wr3 (uint8)'}  outputporttype=[3]  outputportwidth=[1]  outputportlabel={'Status'}  compat=0  optionstring="[\"1\",\"4\",\"0\",\"5\",\"off\",\"1\"]"
  Success : Outport
  wires:
  D1/1 -> Soft I2C Master Read/Write/4
  SlaveAddr/1 -> Soft I2C Master Read/Write/1
  Offset/1 -> Soft I2C Master Read/Write/2
  Soft I2C Master Read/Write/1 -> Compare To Zero/1
  D0/1 -> Soft I2C Master Read/Write/3
  Compare To Zero/1 -> Success/1
  D2/1 -> Soft I2C Master Read/Write/5
